simulink model "asignacion_polos"  (Simulink 5.0)
settings: Solver=ode45  StartTime=0.0  StopTime=5  RelTol=1e-3
undefined symbols (not defined in the file): A, B, Blockset_Practica2, Diseño, ts
libraries: simulink x7, dsparch4 x2
settings Model: LastModifiedBy=pc1

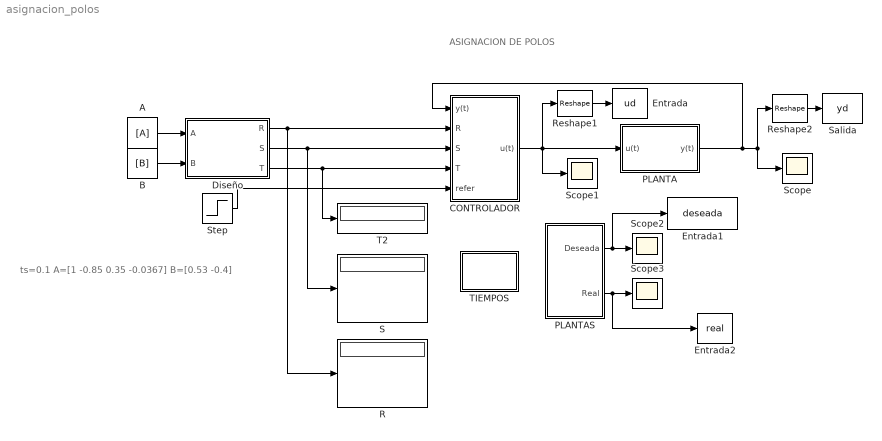
== system asignacion_polos ==
  note: ASIGNACION DE POLOS
  note: ts=0.1
      | A=[1 -0.85 0.35 -0.0367]
      | B=[0.53 -0.4]
  A : Constant  Value=[A]
  B : Constant  Value=[B]
  CONTROLADOR : Subsystem
  Diseño : Subsystem  AncestorBlock=Blockset_Practica2/Diseño  mask{Am=[1 -1.6 .6925 .10475 -.1364 .00242], A0=1}
      mask Display: disp('Diseño')
  Entrada : ToWorkspace  VariableName=ud  SampleTime=ts  SaveFormat=Array
  Entrada1 : ToWorkspace  VariableName=deseada  SampleTime=ts  SaveFormat=Array
  Entrada2 : ToWorkspace  VariableName=real  SampleTime=ts  SaveFormat=Array
  PLANTA : Subsystem
  PLANTAS : Subsystem
  R : Display
  Reshape1 : simulink/Math Operations/Reshape  OutputDimensionality=1-D array  OutputDimensions=[1,1]
  Reshape2 : simulink/Math Operations/Reshape  OutputDimensionality=1-D array  OutputDimensions=[1,1]
  S : Display
  Salida : ToWorkspace  VariableName=yd  SampleTime=ts  SaveFormat=Array
  Scope{,1..3} (4 alike) : Scope
      Scope settings: TimeRange=10  YMin=0  YMax=1.4
      Scope1 settings: TimeRange=10  YMin=0  YMax=1.4  SaveName=ScopeData2
      Scope2 settings: TimeRange=10  YMin=0  YMax=1.4
      Scope3 settings: TimeRange=10  YMin=0  YMax=1.4  SaveName=ScopeData3
  Step : Step  Time=0  SampleTime=0
  T2 : Display
  TIEMPOS : Subsystem
  wires:
  PLANTA/1(y(t)) -> Scope/1, Reshape2/1, CONTROLADOR/1(y(t))
  CONTROLADOR/1(u(t)) -> Scope1/1, PLANTA/1(u(t)), Reshape1/1
  PLANTAS/1(Deseada) -> Scope2/1, Entrada1/1
  PLANTAS/2(Real) -> Scope3/1, Entrada2/1
  Diseño/1(R) -> CONTROLADOR/2(R), R/1
  Diseño/2(S) -> CONTROLADOR/3(S), S/1
  Diseño/3(T) -> CONTROLADOR/4(T), T2/1
  Step/1 -> CONTROLADOR/5(refer)
  A/1 -> Diseño/1(A)
  B/1 -> Diseño/2(B)
  Reshape2/1 -> Salida/1
  Reshape1/1 -> Entrada/1

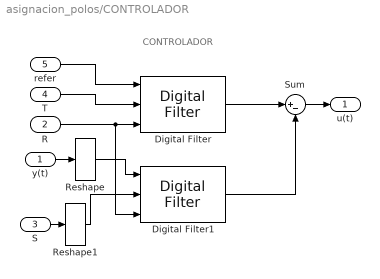
== system asignacion_polos/CONTROLADOR ==
  note: CONTROLADOR
  y(t) : Inport
  R : Inport  Port=2
  S : Inport  Port=3
  T : Inport  Port=4
  refer : Inport  Port=5
  Digital Filter : dsparch4/Digital Filter  TypePopup=IIR (poles & zeros)  IIRFiltStruct=Direct form II  AllPoleFiltStruct=Direct form  FIRFiltStruct=Direct form  CoeffSource=Input port(s)  NumCoeffs=[1 2]  DenCoeffs=[1 0.1]  BiQuadCoeffs=[1 0.3 0.4 1 0.1 0.2]  LatticeCoeffs=[0.2 0.4]  denIgnore=on  FiltPerSampPopup=One filter per frame  IC=0  ICnum=0  ICden=0
  Digital Filter1 : dsparch4/Digital Filter  TypePopup=IIR (poles & zeros)  IIRFiltStruct=Direct form II  AllPoleFiltStruct=Direct form  FIRFiltStruct=Direct form  CoeffSource=Input port(s)  NumCoeffs=[1 2]  DenCoeffs=[1 0.1]  BiQuadCoeffs=[1 0.3 0.4 1 0.1 0.2]  LatticeCoeffs=[0.2 0.4]  denIgnore=on  FiltPerSampPopup=One filter per frame  IC=0  ICnum=0  ICden=0
  Reshape : simulink/Math Operations/Reshape  OutputDimensionality=Column vector  OutputDimensions=[1,1]
  Reshape1 : simulink/Math Operations/Reshape  OutputDimensionality=Column vector  OutputDimensions=[1,1]
  Sum : Sum  Inputs=|+-  SaturateOnIntegerOverflow=on
  u(t) : Outport
  wires:
  Sum/1 -> u(t)/1
  Digital Filter/1 -> Sum/1
  Digital Filter1/1 -> Sum/2
  R/1 -> Digital Filter1/3, Digital Filter/3
  Reshape1/1 -> Digital Filter1/2
  T/1 -> Digital Filter/2
  refer/1 -> Digital Filter/1
  S/1 -> Reshape1/1
  y(t)/1 -> Reshape/1
  Reshape/1 -> Digital Filter1/1

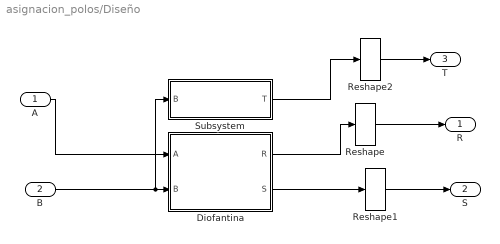
== system asignacion_polos/Diseño ==
  A : Inport
  B : Inport  Port=2
  Diofantina : Subsystem  mask{Ac=conv(Am,A0)}
      mask Display: disp('Diofantica')
  Reshape : simulink/Math Operations/Reshape  OutputDimensionality=Column vector  OutputDimensions=[1,1]
  Reshape1 : simulink/Math Operations/Reshape  OutputDimensionality=Column vector  OutputDimensions=[1,1]
  Reshape2 : simulink/Math Operations/Reshape  OutputDimensionality=Column vector  OutputDimensions=[1,1]
  Subsystem : Subsystem  mask{Am=Am, A0=A0}
      mask Display: disp('Polinomio T')
  R : Outport
  S : Outport  Port=2
  T : Outport  Port=3
  wires:
  Subsystem/1(T) -> Reshape2/1
  Diofantina/1(R) -> Reshape/1
  A/1 -> Diofantina/1(A)
  Diofantina/2(S) -> Reshape1/1
  B/1 -> Diofantina/2(B), Subsystem/1(B)
  Reshape/1 -> R/1
  Reshape1/1 -> S/1
  Reshape2/1 -> T/1

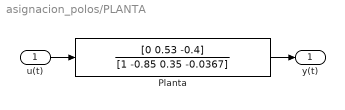
== system asignacion_polos/PLANTA ==
  u(t) : Inport
  Planta : DiscreteFilter  Numerator=[0 0.53 -0.4]  Denominator=[1 -0.85 0.35 -0.0367]  SampleTime=.1
  y(t) : Outport
  wires:
  u(t)/1 -> Planta/1
  Planta/1 -> y(t)/1

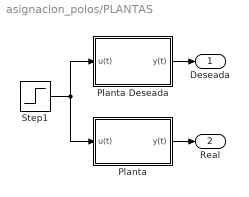
== system asignacion_polos/PLANTAS ==
  Planta : Subsystem
  Planta Deseada : Subsystem  mask{Bm=[0.5300   -0.4000]*.4867, Am=[1 -1.6 .6925 .10475 -.1364 .00242], ts=ts}
      mask prompts: Bm "Polinomio Numerador Bm"; Am "Polinomio Denominador Am"; ts "Tiempo de Muestreo"
  Step1 : Step  Time=0  SampleTime=0
  Deseada : Outport
  Real : Outport  Port=2
  wires:
  Step1/1 -> Planta Deseada/1(u(t)), Planta/1(u(t))
  Planta Deseada/1(y(t)) -> Deseada/1
  Planta/1(y(t)) -> Real/1

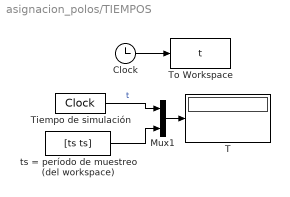
== system asignacion_polos/TIEMPOS ==
  Clock : Clock
      settings: Decimation=10
  Mux1 : Mux  Inputs=2
  T : Display
  Tiempo de simulación : DigitalClock  SampleTime=.1
  To Workspace : ToWorkspace  VariableName=t  SampleTime=ts  SaveFormat=Array
  ts = período de muestreo (del workspace) : FromWorkspace  VariableName=[ts ts]  SampleTime=0
  wires:
  Clock/1 -> To Workspace/1
  ts = período de muestreo (del workspace)/1 -> Mux1/2
  Tiempo de simulación/1 -> Mux1/1  "t"
  Mux1/1 -> T/1

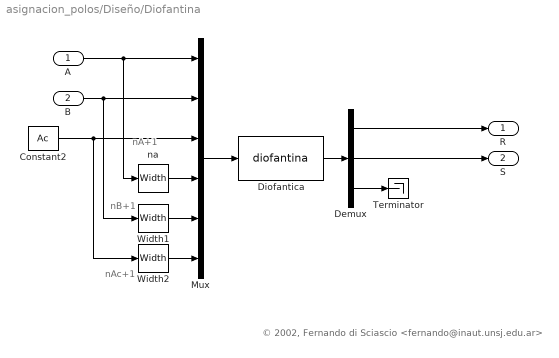
== system asignacion_polos/Diseño/Diofantina ==
  note: nAc+1
  note: nA+1
  note: nB+1
  note: © 2002, Fernando di Sciascio <fernando@inaut.unsj.edu.ar>
  A : Inport
  B : Inport  Port=2
  Constant2 : Constant  Value=Ac
  Demux : Demux  Outputs="[length(Ac)-length(A)+1  length(A)-1  length(A)+length(B)+length(Ac) - (length(Ac)-length(A)+1) -  ( length(A)-1 )+3]"
  Diofantica : S-Function  FunctionName=diofantina
      mask Type: S-function: timestwo
      mask Description: Esta S-function resuelve la ecuacion diofantina
      mask Help:
      | Dados los polinomios A, B, Ac y los ordenes de los polinomios R y S esta
      | S-function resuelve la ecuacion diofantina:
      | 
      |     A*R+B*S=Ac
      mask Display: disp('        Diofantina      ');
  Mux : Mux  Inputs=6
  Terminator : Terminator
  Width1 : Width
  Width2 : Width
  na : Width
  R : Outport
  S : Outport  Port=2
  wires:
  Mux/1 -> Diofantica/1
  Constant2/1 -> Mux/3, Width2/1
  Diofantica/1 -> Demux/1
  Demux/3 -> Terminator/1
  A/1 -> Mux/1, na/1
  B/1 -> Mux/2, Width1/1
  Demux/1 -> R/1
  Demux/2 -> S/1
  na/1 -> Mux/4
  Width1/1 -> Mux/5
  Width2/1 -> Mux/6

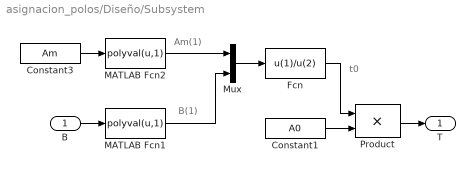
== system asignacion_polos/Diseño/Subsystem ==
  note: B(1)
  note: Am(1)
  note: t0
  B : Inport
  Constant1 : Constant  Value=A0
  Constant3 : Constant  Value=Am
  Fcn : Fcn  Expr=u(1)/u(2)
  MATLAB Fcn1 : MATLABFcn  MATLABFcn=polyval(u,1)
  MATLAB Fcn2 : MATLABFcn  MATLABFcn=polyval(u,1)
  Mux : Mux  Inputs=2
  Product : Product  SaturateOnIntegerOverflow=on  InputSameDT=on
  T : Outport
  wires:
  Mux/1 -> Fcn/1
  MATLAB Fcn2/1 -> Mux/1
  MATLAB Fcn1/1 -> Mux/2
  Fcn/1 -> Product/1
  Constant3/1 -> MATLAB Fcn2/1
  Product/1 -> T/1
  B/1 -> MATLAB Fcn1/1
  Constant1/1 -> Product/2

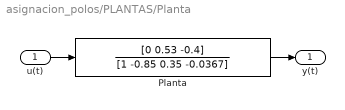
== system asignacion_polos/PLANTAS/Planta ==
  u(t) : Inport
  Planta : DiscreteFilter  Numerator=[0 0.53 -0.4]  Denominator=[1 -0.85 0.35 -0.0367]  SampleTime=.1
  y(t) : Outport
  wires:
  u(t)/1 -> Planta/1
  Planta/1 -> y(t)/1

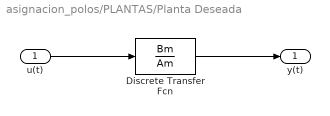
== system asignacion_polos/PLANTAS/Planta Deseada ==
  u(t) : Inport
  Discrete Transfer Fcn : DiscreteTransferFcn  Numerator=Bm  Denominator=Am  SampleTime=ts
  y(t) : Outport
  wires:
  u(t)/1 -> Discrete Transfer Fcn/1
  Discrete Transfer Fcn/1 -> y(t)/1
